simulink model "IEEE9bus"  (R2023a)
settings: Solver=VariableStepAuto  StartTime=0.0  StopTime=10.0  RelTol=1e-3
libraries: spsThreePhaseVIMeasurementLib x11, spsDistributedParametersLineLib x9, spsThreePhaseBreakerLib x9, spsThreePhaseTransformerTwoWindingsLib x6, eePMU x4, spsThreePhaseSourceLib x3, spsThreePhaseParallelRLCLoadLib x3, spsThreePhaseFaultLib x2
settings Model: Creator=Pranesh  LastModifiedBy=Pranesh

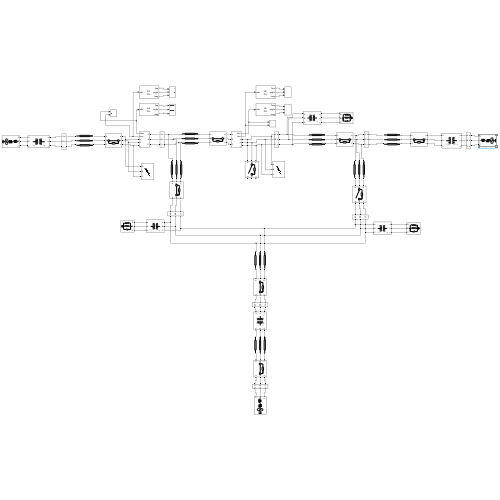
[thumbnail: Simulink's stored preview of the top-level diagram]
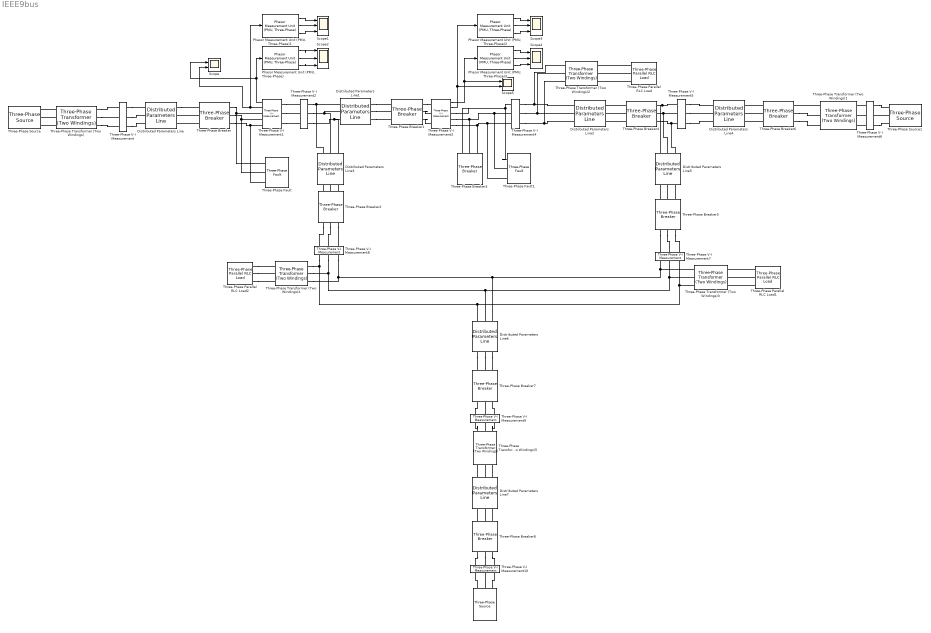
== system IEEE9bus ==
  " " : spsThreePhaseSourceLib/Three-Phase Source  InternalConnection=Yg  VoltagePhases=off  Voltage=25e3  PhaseAngle=0  Voltage_phases=[25e3 25e3 25e3]/sqrt(3)  PhaseAngles_phases=[0 -120 +120]  Frequency=60  NonIdealSource=on  SpecifyImpedance=off  Resistance=0.8929  Inductance=16.58e-3  ShortCircuitLevel=100e6  BaseVoltage=25e3  XRratio=7  BusType=swing  Pref=10e3  Qref=0  Prefabc=[10e3, 10e3, 10e3]  Qrefabc=[0, 0, 0]  Qmin=-inf  Qmax=inf
  "  " : spsDistributedParametersLineLib/Distributed Parameters Line  Phases=3  Length=100  Frequency=60  Resistance=[0.01273 0.3864]  Inductance="[0.9337e-3  4.1264e-3]"  Capacitance=[12.74e-9 7.751e-9]  x1=[0 0 0 0; 0.0001244 0 0 0; 0.0002488 0 0 0; 0.0003733 0 0 0; 0.0004977 0 0 0; 0.0006221 0 0 0]  x2=[0 0 0 0; 0.0001244 0 0 0; 0.0002488 0 0 0; 0.0003733 0 0 0; 0.0004977 0 0 0; 0.0006221 0 0 0]  x3=[0 0 0 0; 0.0001244 0 0 0; 0.0002488 0 0 0; 0.0003733 0 0 0; 0.0004977 0 0 0; 0.0006221 0 0 0]  x4=[0 0 0 0; 0.0001244 0 0 0; 0.0002488 0 0 0; 0.0003733 0 0 0; 0.0004977 0 0 0; 0.0006221 0 0 0]  x5=0  V1=ones(3,3)  V2=ones(3,3)  I1=ones(3,3)  I2=ones(3,3)  nHarmo=1  Measurements=None  Decoupling=off  VsMag0=0  VrMag0=0  VsAngle0=0  VrAngle0=0  IsMag0=0  IrMag0=0  IsAngle0=0  IrAngle0=0
      settings: LibrarySourceBlock=sps_lib/Power Grid Elements/Distributed Parameters Line
  Distributed Parameters Line{,1..7} (8 alike) : spsDistributedParametersLineLib/Distributed Parameters Line  Phases=3  Length=100  Frequency=60  Resistance=[0.01273 0.3864]  Inductance="[0.9337e-3  4.1264e-3]"  Capacitance=[12.74e-9 7.751e-9]  x1=[0 0 0 0; 0.0001244 0 0 0; 0.0002488 0 0 0; 0.0003733 0 0 0; 0.0004977 0 0 0; 0.0006221 0 0 0]  x2=[0 0 0 0; 0.0001244 0 0 0; 0.0002488 0 0 0; 0.0003733 0 0 0; 0.0004977 0 0 0; 0.0006221 0 0 0]  x3=[0 0 0 0; 0.0001244 0 0 0; 0.0002488 0 0 0; 0.0003733 0 0 0; 0.0004977 0 0 0; 0.0006221 0 0 0]  x4=[0 0 0 0; 0.0001244 0 0 0; 0.0002488 0 0 0; 0.0003733 0 0 0; 0.0004977 0 0 0; 0.0006221 0 0 0]  x5=0  V1=ones(3,3)  V2=ones(3,3)  I1=ones(3,3)  I2=ones(3,3)  nHarmo=1  Measurements=None  Decoupling=off  VsMag0=0  VrMag0=0  VsAngle0=0  VrAngle0=0  IsMag0=0  IrMag0=0  IsAngle0=0  IrAngle0=0
      settings: LibrarySourceBlock=sps_lib/Power Grid Elements/Distributed Parameters Line
  Phasor Measurement Unit (PMU, Three-Phase){,1..3} (4 alike) : eePMU/Phasor Measurement Unit (PMU, Three-Phase)  frequency=60  Nsr=64  k=1
      settings: LibrarySourceBlock=|
      | ee_sl_lib/Measurements/Phasor Measurement Unit
      | (PMU, Three-Phase)
  Scope : Scope  NumInputPorts=2
  Scope{1..4} (4 alike) : Scope  NumInputPorts=3
  Scope5 : Scope  NumInputPorts=2
  Three-Phase Parallel RLC Load : spsThreePhaseParallelRLCLoadLib/Three-Phase Parallel RLC Load  LConnTagsString=A|B|C  Configuration=Y (grounded)  NominalVoltage=1000  Vabc=[1e3 1e3 1e3]  Vabcp=[1e3 1e3 1e3]  NominalFrequency=60  UnbalancedPower=off  ActivePower=10e3  InductivePower=100  CapacitivePower=100  Pabc=[10e3 9e3 11e3]  QLabc=[100 90 110]  QCabc=[100 90 110]  Pabcp=[10e3 9e3 11e3]  QLabcp=[100 90 110]  QCabcp=[100 90 110]  Measurements=None  LoadType=constant Z
  Three-Phase Parallel RLC Load1 : spsThreePhaseParallelRLCLoadLib/Three-Phase Parallel RLC Load  LConnTagsString=A|B|C  Configuration=Y (grounded)  NominalVoltage=1000  Vabc=[1e3 1e3 1e3]  Vabcp=[1e3 1e3 1e3]  NominalFrequency=60  UnbalancedPower=off  ActivePower=10e3  InductivePower=100  CapacitivePower=100  Pabc=[10e3 9e3 11e3]  QLabc=[100 90 110]  QCabc=[100 90 110]  Pabcp=[10e3 9e3 11e3]  QLabcp=[100 90 110]  QCabcp=[100 90 110]  Measurements=None  LoadType=constant Z
  Three-Phase Parallel RLC Load2 : spsThreePhaseParallelRLCLoadLib/Three-Phase Parallel RLC Load  LConnTagsString=A|B|C  Configuration=Y (grounded)  NominalVoltage=1000  Vabc=[1e3 1e3 1e3]  Vabcp=[1e3 1e3 1e3]  NominalFrequency=60  UnbalancedPower=off  ActivePower=10e3  InductivePower=100  CapacitivePower=100  Pabc=[10e3 9e3 11e3]  QLabc=[100 90 110]  QCabc=[100 90 110]  Pabcp=[10e3 9e3 11e3]  QLabcp=[100 90 110]  QCabcp=[100 90 110]  Measurements=None  LoadType=constant Z
  Three-Phase Transformer (Two Windings){,1..5} (6 alike) : spsThreePhaseTransformerTwoWindingsLib/Three-Phase Transformer (Two Windings)  Winding1Connection=Yg  Winding2Connection=Yg  CoreType=Three single-phase transformers  SetSaturation=off  Hysteresis=off  DataFile='hysteresis'  SetInitialFlux=off  Measurements=None  UNITS=pu  NominalPower=[ 250e6 , 60 ]  Winding1=[ 735e3 , 0.002 , 0.08 ]  Winding2=[ 315e3 , 0.002 , 0.08 ]  Rm=500  Lm=500  L0=0.5  Saturation=[ 0,0 ; 0.0024,1.2 ; 1.0,1.52 ]  InitialFluxes=[ 0.8 , -0.8 , 0.7 ]  BreakLoop=off  DiscreteSolver=Trapezoidal iterative  DataType=off  TransfoNumber=1
  Three-Phase V-I Measurement : spsThreePhaseVIMeasurementLib/Three-Phase V-I Measurement  VoltageMeasurement=phase-to-ground  SetLabelV=on  LabelV=Vbus_2  Vpu=off  VpuLL=off  CurrentMeasurement=yes  SetLabelI=on  LabelI=Ibus_2  Ipu=off  Pbase=100e6  Vbase=500e3  OutputType=Complex  PhasorSimulation=off  PSBequivalent=0
  Three-Phase V-I Measurement1 : spsThreePhaseVIMeasurementLib/Three-Phase V-I Measurement  VoltageMeasurement=phase-to-ground  SetLabelV=off  LabelV=Vabc  Vpu=off  VpuLL=off  CurrentMeasurement=yes  SetLabelI=off  LabelI=Iabc  Ipu=off  Pbase=100e6  Vbase=500e3  OutputType=Complex  PhasorSimulation=off  PSBequivalent=0
  Three-Phase V-I Measurement{2,4..10} (8 alike) : spsThreePhaseVIMeasurementLib/Three-Phase V-I Measurement  VoltageMeasurement=phase-to-ground  SetLabelV=on  LabelV=Vbus_7  Vpu=off  VpuLL=off  CurrentMeasurement=yes  SetLabelI=on  LabelI=Ibus_7  Ipu=off  Pbase=100e6  Vbase=500e3  OutputType=Complex  PhasorSimulation=off  PSBequivalent=0
  Three-Phase V-I Measurement3 : spsThreePhaseVIMeasurementLib/Three-Phase V-I Measurement  VoltageMeasurement=phase-to-ground  SetLabelV=off  LabelV=Vabc  Vpu=off  VpuLL=off  CurrentMeasurement=yes  SetLabelI=off  LabelI=Iabc  Ipu=off  Pbase=100e6  Vbase=500e3  OutputType=Complex  PhasorSimulation=off  PSBequivalent=0
  Three-Phase Breaker{,1..2,4,6..8} (7 alike) : spsThreePhaseBreakerLib/Three-Phase Breaker  InitialState=closed  SwitchA=on  SwitchB=on  SwitchC=on  SwitchTimes="[1/60  5/60]"  External=off  BreakerResistance=0.01  SnubberResistance=1e6  SnubberCapacitance=inf  Measurements=None
  Three-Phase Breaker3 : spsThreePhaseBreakerLib/Three-Phase Breaker  InitialState=open  SwitchA=on  SwitchB=on  SwitchC=on  SwitchTimes="[1/60  5/60]"  External=off  BreakerResistance=0.01  SnubberResistance=1e6  SnubberCapacitance=inf  Measurements=None
  Three-Phase Breaker5 : spsThreePhaseBreakerLib/Three-Phase Breaker  InitialState=open  SwitchA=on  SwitchB=on  SwitchC=on  SwitchTimes="[1/60  5/60]"  External=off  BreakerResistance=0.01  SnubberResistance=1e6  SnubberCapacitance=inf  Measurements=None
  Three-Phase Fault : spsThreePhaseFaultLib/Three-Phase Fault  InitialStates=0  FaultA=on  FaultB=on  FaultC=on  GroundFault=on  SwitchTimes="[1/60  5/60]"  External=off  SwitchStatus=NaN  FaultResistance=0.001  GroundResistance=0.01  SnubberResistance=1e6  SnubberCapacitance=inf  Measurements=None
  Three-Phase Fault1 : spsThreePhaseFaultLib/Three-Phase Fault  InitialStates=0  FaultA=on  FaultB=on  FaultC=on  GroundFault=on  SwitchTimes="[1/60  5/60]"  External=off  SwitchStatus=NaN  FaultResistance=0.001  GroundResistance=0.01  SnubberResistance=1e6  SnubberCapacitance=inf  Measurements=None
  Three-Phase Source : spsThreePhaseSourceLib/Three-Phase Source  InternalConnection=Yg  VoltagePhases=off  Voltage=25e3  PhaseAngle=0  Voltage_phases=[25e3 25e3 25e3]/sqrt(3)  PhaseAngles_phases=[0 -120 +120]  Frequency=60  NonIdealSource=on  SpecifyImpedance=off  Resistance=0.8929  Inductance=16.58e-3  ShortCircuitLevel=100e6  BaseVoltage=25e3  XRratio=7  BusType=swing  Pref=10e3  Qref=0  Prefabc=[10e3, 10e3, 10e3]  Qrefabc=[0, 0, 0]  Qmin=-inf  Qmax=inf
  Three-Phase Source1 : spsThreePhaseSourceLib/Three-Phase Source  InternalConnection=Yg  VoltagePhases=off  Voltage=25e3  PhaseAngle=0  Voltage_phases=[25e3 25e3 25e3]/sqrt(3)  PhaseAngles_phases=[0 -120 +120]  Frequency=60  NonIdealSource=on  SpecifyImpedance=off  Resistance=0.8929  Inductance=16.58e-3  ShortCircuitLevel=100e6  BaseVoltage=25e3  XRratio=7  BusType=swing  Pref=10e3  Qref=0  Prefabc=[10e3, 10e3, 10e3]  Qrefabc=[0, 0, 0]  Qmin=-inf  Qmax=inf
  wires:
  "Phasor Measurement Unit (PMU, Three-Phase)"/1 -> Scope2/1
  "Phasor Measurement Unit (PMU, Three-Phase)"/2 -> Scope2/2
  "Phasor Measurement Unit (PMU, Three-Phase)"/3 -> Scope2/3
  "Phasor Measurement Unit (PMU, Three-Phase)1"/1 -> Scope1/1
  "Phasor Measurement Unit (PMU, Three-Phase)1"/2 -> Scope1/2
  "Phasor Measurement Unit (PMU, Three-Phase)1"/3 -> Scope1/3
  Three-Phase V-I Measurement1/1 -> Scope/1, "Phasor Measurement Unit (PMU, Three-Phase)"/1
  Three-Phase V-I Measurement1/2 -> "Phasor Measurement Unit (PMU, Three-Phase)1"/1, Scope/2
  "Phasor Measurement Unit (PMU, Three-Phase)3"/2 -> Scope4/2
  "Phasor Measurement Unit (PMU, Three-Phase)3"/3 -> Scope4/3
  "Phasor Measurement Unit (PMU, Three-Phase)3"/1 -> Scope4/1
  "Phasor Measurement Unit (PMU, Three-Phase)2"/3 -> Scope3/3
  "Phasor Measurement Unit (PMU, Three-Phase)2"/2 -> Scope3/2
  "Phasor Measurement Unit (PMU, Three-Phase)2"/1 -> Scope3/1
  Three-Phase V-I Measurement3/1 -> Scope5/1, "Phasor Measurement Unit (PMU, Three-Phase)3"/1
  Three-Phase V-I Measurement3/2 -> Scope5/2, "Phasor Measurement Unit (PMU, Three-Phase)2"/1
  connections:
  Three-Phase Transformer (Two Windings)/LConn3 -- Three-Phase Source/RConn3
  Three-Phase Transformer (Two Windings)/LConn2 -- Three-Phase Source/RConn2
  Three-Phase Transformer (Two Windings)/LConn1 -- Three-Phase Source/RConn1
  Three-Phase Transformer (Two Windings)/RConn2 -- Three-Phase V-I Measurement/LConn2
  Three-Phase Transformer (Two Windings)/RConn3 -- Three-Phase V-I Measurement/LConn3
  Three-Phase Transformer (Two Windings)/RConn1 -- Three-Phase V-I Measurement/LConn1
  Three-Phase V-I Measurement/RConn2 -- Distributed Parameters Line/LConn2
  Three-Phase V-I Measurement/RConn3 -- Distributed Parameters Line/LConn3
  Three-Phase V-I Measurement/RConn1 -- Distributed Parameters Line/LConn1
  Three-Phase Breaker/LConn3 -- Distributed Parameters Line/RConn3
  Three-Phase Breaker/LConn2 -- Distributed Parameters Line/RConn2
  Distributed Parameters Line/RConn1 -- Three-Phase Breaker/LConn1
  Three-Phase Breaker/RConn3 -- Three-Phase Fault/LConn3 -- Three-Phase V-I Measurement1/RConn3
  Three-Phase Breaker/RConn1 -- Three-Phase V-I Measurement1/RConn1 -- Three-Phase Fault/LConn1
  Three-Phase Breaker/RConn2 -- Three-Phase V-I Measurement1/RConn2 -- Three-Phase Fault/LConn2
  Three-Phase V-I Measurement1/LConn1 -- Three-Phase V-I Measurement2/LConn1
  Three-Phase V-I Measurement1/LConn2 -- Three-Phase V-I Measurement2/LConn2
  Three-Phase V-I Measurement1/LConn3 -- Three-Phase V-I Measurement2/LConn3
  Three-Phase V-I Measurement2/RConn2 -- "  "/RConn2 -- Distributed Parameters Line1/LConn2
  Three-Phase V-I Measurement2/RConn1 -- "  "/RConn1 -- Distributed Parameters Line1/LConn1
  Three-Phase V-I Measurement2/RConn3 -- Distributed Parameters Line3/RConn3 -- Distributed Parameters Line1/LConn3
  Distributed Parameters Line1/RConn1 -- Three-Phase Breaker1/LConn1
  Distributed Parameters Line1/RConn2 -- Three-Phase Breaker1/LConn2
  Distributed Parameters Line1/RConn3 -- Three-Phase Breaker1/LConn3
  Three-Phase Breaker2/LConn1 -- Distributed Parameters Line3/LConn1
  Three-Phase Breaker2/LConn2 -- Distributed Parameters Line3/LConn2
  Three-Phase Breaker2/LConn3 -- Distributed Parameters Line3/LConn3
  Three-Phase Breaker1/RConn2 -- Three-Phase V-I Measurement3/LConn2
  Three-Phase Breaker1/RConn3 -- Three-Phase V-I Measurement3/LConn3
  Three-Phase Breaker1/RConn1 -- Three-Phase V-I Measurement3/LConn1
  Three-Phase Fault1/LConn1 -- Three-Phase V-I Measurement3/RConn1 -- Three-Phase Breaker3/LConn1 -- Three-Phase V-I Measurement4/LConn1
  Three-Phase V-I Measurement3/RConn2 -- Three-Phase Breaker3/LConn2 -- Three-Phase Fault1/LConn2 -- Three-Phase V-I Measurement4/LConn2
  Three-Phase V-I Measurement3/RConn3 -- Three-Phase Breaker3/LConn3 -- Three-Phase Fault1/LConn3 -- Three-Phase V-I Measurement4/LConn3
  Three-Phase V-I Measurement4/RConn1 -- Three-Phase Transformer (Two Windings)2/LConn1 -- Distributed Parameters Line2/LConn1
  Three-Phase V-I Measurement4/RConn2 -- Three-Phase Transformer (Two Windings)2/LConn2 -- Distributed Parameters Line2/LConn2
  Three-Phase V-I Measurement4/RConn3 -- Three-Phase Transformer (Two Windings)2/LConn3 -- Distributed Parameters Line2/LConn3
  Three-Phase Breaker4/LConn3 -- Distributed Parameters Line2/RConn3
  Three-Phase Breaker4/LConn2 -- Distributed Parameters Line2/RConn2
  Three-Phase Breaker4/LConn1 -- Distributed Parameters Line2/RConn1
  Three-Phase V-I Measurement5/LConn2 -- Distributed Parameters Line5/RConn2 -- Three-Phase Breaker4/RConn2
  Three-Phase Breaker4/RConn1 -- Three-Phase V-I Measurement5/LConn1 -- Distributed Parameters Line5/RConn1
  Three-Phase Breaker4/RConn3 -- Distributed Parameters Line5/RConn3 -- Three-Phase V-I Measurement5/LConn3
  Three-Phase V-I Measurement5/RConn3 -- Distributed Parameters Line4/LConn3
  Three-Phase V-I Measurement5/RConn2 -- Distributed Parameters Line4/LConn2
  Three-Phase V-I Measurement5/RConn1 -- Distributed Parameters Line4/LConn1
  Three-Phase Breaker6/LConn3 -- Distributed Parameters Line4/RConn3
  Three-Phase Breaker6/LConn2 -- Distributed Parameters Line4/RConn2
  Three-Phase Breaker6/LConn1 -- Distributed Parameters Line4/RConn1
  Three-Phase Transformer (Two Windings)1/LConn1 -- Three-Phase Breaker6/RConn1
  Three-Phase Breaker6/RConn2 -- Three-Phase Transformer (Two Windings)1/LConn2
  Three-Phase Breaker6/RConn3 -- Three-Phase Transformer (Two Windings)1/LConn3
  Three-Phase V-I Measurement6/LConn3 -- Three-Phase Transformer (Two Windings)1/RConn3
  Three-Phase V-I Measurement6/LConn2 -- Three-Phase Transformer (Two Windings)1/RConn2
  Three-Phase V-I Measurement6/LConn1 -- Three-Phase Transformer (Two Windings)1/RConn1
  Three-Phase Source1/RConn2 -- Three-Phase V-I Measurement6/RConn2
  Three-Phase V-I Measurement6/RConn1 -- Three-Phase Source1/RConn1
  Three-Phase V-I Measurement6/RConn3 -- Three-Phase Source1/RConn3
  Three-Phase Breaker5/LConn1 -- Distributed Parameters Line5/LConn1
  Three-Phase Breaker5/LConn2 -- Distributed Parameters Line5/LConn2
  Three-Phase Breaker5/LConn3 -- Distributed Parameters Line5/LConn3
  Three-Phase Breaker5/RConn3 -- Three-Phase V-I Measurement7/LConn3
  Three-Phase Breaker5/RConn2 -- Three-Phase V-I Measurement7/LConn2
  Three-Phase Breaker5/RConn1 -- Three-Phase V-I Measurement7/LConn1
  Three-Phase Breaker2/RConn3 -- Three-Phase V-I Measurement8/LConn3
  Three-Phase Breaker2/RConn2 -- Three-Phase V-I Measurement8/LConn2
  Three-Phase Breaker2/RConn1 -- Three-Phase V-I Measurement8/LConn1
  Three-Phase V-I Measurement8/RConn3 -- Three-Phase Transformer (Two Windings)4/LConn3 -- Distributed Parameters Line6/RConn3 -- Three-Phase Transformer (Two Windings)3/LConn1 -- Three-Phase V-I Measurement7/RConn1
  Three-Phase V-I Measurement8/RConn2 -- Three-Phase Transformer (Two Windings)4/LConn2 -- Distributed Parameters Line6/RConn2 -- Three-Phase Transformer (Two Windings)3/LConn2 -- Three-Phase V-I Measurement7/RConn2
  Three-Phase V-I Measurement8/RConn1 -- Three-Phase Transformer (Two Windings)4/LConn1 -- Distributed Parameters Line6/RConn1 -- Three-Phase Transformer (Two Windings)3/LConn3 -- Three-Phase V-I Measurement7/RConn3
  Distributed Parameters Line6/LConn1 -- Three-Phase Breaker7/LConn1
  Distributed Parameters Line6/LConn2 -- Three-Phase Breaker7/LConn2
  Distributed Parameters Line6/LConn3 -- Three-Phase Breaker7/LConn3
  Distributed Parameters Line7/RConn1 -- Three-Phase Transformer (Two Windings)5/LConn1
  Distributed Parameters Line7/RConn2 -- Three-Phase Transformer (Two Windings)5/LConn2
  Distributed Parameters Line7/RConn3 -- Three-Phase Transformer (Two Windings)5/LConn3
  Three-Phase Breaker8/LConn1 -- Distributed Parameters Line7/LConn1
  Three-Phase Breaker8/LConn2 -- Distributed Parameters Line7/LConn2
  Three-Phase Breaker8/LConn3 -- Distributed Parameters Line7/LConn3
  Three-Phase V-I Measurement9/LConn1 -- Three-Phase Breaker7/RConn1
  Three-Phase V-I Measurement9/LConn2 -- Three-Phase Breaker7/RConn2
  Three-Phase V-I Measurement9/LConn3 -- Three-Phase Breaker7/RConn3
  Three-Phase Transformer (Two Windings)5/RConn2 -- Three-Phase V-I Measurement9/RConn2
  Three-Phase Transformer (Two Windings)5/RConn3 -- Three-Phase V-I Measurement9/RConn3
  Three-Phase Transformer (Two Windings)5/RConn1 -- Three-Phase V-I Measurement9/RConn1
  Three-Phase Breaker8/RConn1 -- Three-Phase V-I Measurement10/LConn1
  Three-Phase Breaker8/RConn2 -- Three-Phase V-I Measurement10/LConn2
  Three-Phase Breaker8/RConn3 -- Three-Phase V-I Measurement10/LConn3
  " "/RConn1 -- Three-Phase V-I Measurement10/RConn1
  " "/RConn2 -- Three-Phase V-I Measurement10/RConn2
  " "/RConn3 -- Three-Phase V-I Measurement10/RConn3
  Three-Phase Parallel RLC Load/LConn3 -- Three-Phase Transformer (Two Windings)2/RConn3
  Three-Phase Parallel RLC Load/LConn2 -- Three-Phase Transformer (Two Windings)2/RConn2
  Three-Phase Parallel RLC Load/LConn1 -- Three-Phase Transformer (Two Windings)2/RConn1
  Three-Phase Parallel RLC Load1/LConn3 -- Three-Phase Transformer (Two Windings)3/RConn3
  Three-Phase Parallel RLC Load1/LConn2 -- Three-Phase Transformer (Two Windings)3/RConn2
  Three-Phase Parallel RLC Load1/LConn1 -- Three-Phase Transformer (Two Windings)3/RConn1
  Three-Phase Parallel RLC Load2/LConn3 -- Three-Phase Transformer (Two Windings)4/RConn3
  Three-Phase Parallel RLC Load2/LConn2 -- Three-Phase Transformer (Two Windings)4/RConn2
  Three-Phase Parallel RLC Load2/LConn1 -- Three-Phase Transformer (Two Windings)4/RConn1
